simulink model "FourierSynthesizer"  (Simulink 7.9)
settings: Solver=ode45  StartTime=0.0  StopTime=100.0  RelTol=1e-3
libraries: simulink_extras x1
settings Model: Creator=Andrew  LastModifiedBy=Andrew

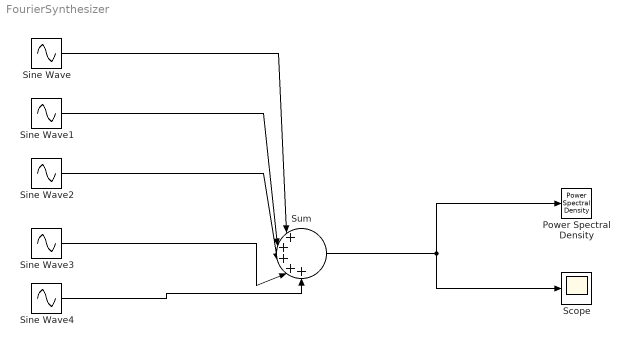
== system FourierSynthesizer ==
  Power Spectral Density : simulink_extras/Additional Sinks/Power Spectral Density  npts=128  fftpts=512  HowOften=64  sampleT=0.1
  Scope : Scope
  Sine Wave : Sin  Amplitude=0.4456  Frequency=.1592  SampleTime=0
  Sine Wave1 : Sin  Amplitude=0.1485  Frequency=0.4775  SampleTime=0
  Sine Wave2 : Sin  Amplitude=0.0891  Frequency=0.7958  SampleTime=0
  Sine Wave3 : Sin  Amplitude=0.0637  Frequency=1.1141  SampleTime=0
  Sine Wave4 : Sin  Amplitude=0.0495  Frequency=1.4324  SampleTime=0
  Sum : Sum  Inputs=|+++++
  wires:
  Sine Wave/1 -> Sum/1
  Sine Wave1/1 -> Sum/2
  Sine Wave2/1 -> Sum/3
  Sine Wave3/1 -> Sum/4
  Sine Wave4/1 -> Sum/5
  Sum/1 -> Power Spectral Density/1, Scope/1
